simulink model "Multmeter"  (R2023b)
settings: Solver=VariableStepAuto  StartTime=0.0  StopTime=10.0  RelTol=1e-3
settings Model: Creator=user  LastModifiedBy=user

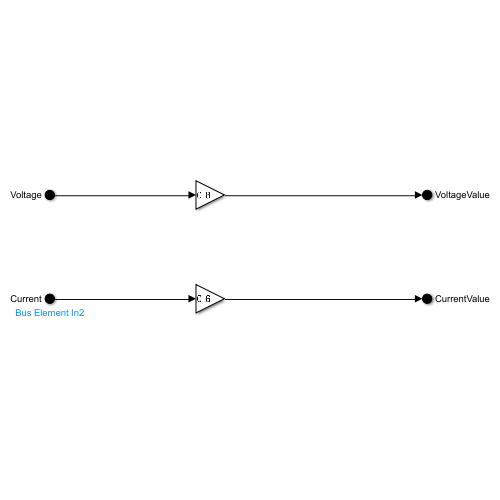
[thumbnail: Simulink's stored preview of the top-level diagram]
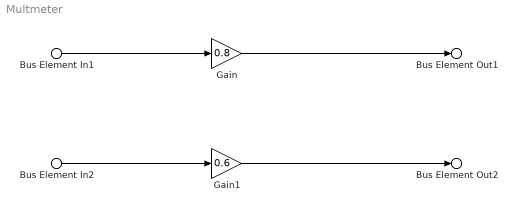
== system Multmeter ==
  Bus Element In1 : Inport  PortName=Voltage
  Bus Element In2 : Inport  Port=2  PortName=Current
  Gain : Gain  Gain=0.8
  Gain1 : Gain  Gain=0.6
  Bus Element Out1 : Outport  PortName=VoltageValue
  Bus Element Out2 : Outport  Port=2  PortName=CurrentValue
  wires:
  Bus Element In1/1 -> Gain/1
  Gain/1 -> Bus Element Out1/1
  Bus Element In2/1 -> Gain1/1
  Gain1/1 -> Bus Element Out2/1
